simulink model "mdaqdemo_external_mode"  (R2014a)
settings: Solver=FixedStepDiscrete  SolverMode=SingleTasking  StartTime=0.0  StopTime=inf  FixedStep=0.001  RelTol=1e-3
libraries: simulink x2, microdaq_lib x2
settings Model: SimulationMode=external  CovSFcnEnable=on  ExtModeTrigDuration=10000  Creator=peselnikmg  LastModifiedBy=skibool
settings DataIOCC: SignalLoggingSaveFormat=ModelDataLogs
settings OptimizationCC: OptimizeModelRefInitCode=on  LifeSpan=1
settings DebuggingCC: UnderspecifiedInitializationDetection=Classic  MultiTaskDSMMsg=warning  MultiTaskCondExecSysMsg=none  FrameProcessingCompatibilityMsg=error  StateNameClashWarn=warning
settings HardwareCC: ProdBitPerLong=40  ProdLargestAtomicInteger=Integer  ProdIntDivRoundTo=Zero  ProdEndianess=LittleEndian  ProdHWDeviceType=Texas Instruments->C6000
settings RTWCC: SystemTargetFile=microdaq.tlc  TemplateMakefile=microdaq.tmf  PostCodeGenCommand=microdaq_postcodegen(buildInfo)  Description=MicroDAQ Real-Time Measurement System  GenerateReport=on  IncludeHyperlinkInReport=on
settings CodeAppCC: IgnoreCustomStorageClasses=off
settings STFCustomTargetCC: CodeReplacementLibrary=C89/C90 (ANSI)  ConcurrentExecutionCompliant=off  GeneratePreprocessorConditionals=Use local settings  CombineOutputUpdateFcns=on  ERTCustomFileBanners=on  SupportContinuousTime=off  SupportNonInlinedSFcns=off  MATLABClassNameForMDSCustomization=Simulink.SoftwareTarget.ERTCustomization  GRTInterface=off  SystemTargetFile=microdaq.tlc
settings ERTTargetCC: CodeReplacementLibrary=C89/C90 (ANSI)  GenerateSampleERTMain=off  ExtMode=on  ExtModeMexArgs=getpref('microdaq','TargetIP') 1 4344  InlinedParameterPlacement=Hierarchical  ERTCustomFileTemplate=microdaq_main.tlc

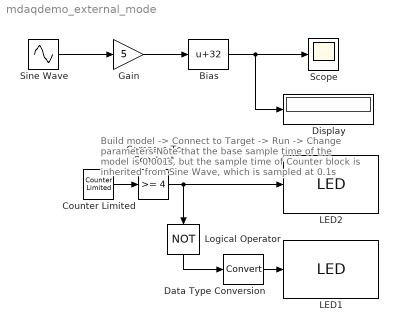
== system mdaqdemo_external_mode ==
  note: Build model -> Connect to Target -> Run -> Change parameters
      |
      | Note that the base sample time of the model is 0.001s,
      | but the sample time of Counter block is inherited from Sine Wave,
      | which is sampled at 0.1s
  Bias : Bias  Bias=32
  Compare To Constant : simulink/Logic and Bit Operations/Compare To Constant  relop=>=  const=4  OutDataTypeStr=uint8
  Counter Limited : simulink/Sources/Counter Limited  uplimit=7  tsamp=-1
      settings: AttributesFormatString=Upper limit: %<uplimit>
  Data Type Conversion : DataTypeConversion
  Display : Display
  Gain : Gain  Gain=5
  LED1 : microdaq_lib/Utilities/LED  SParameter1=D2
  LED2 : microdaq_lib/Utilities/LED  SParameter1=D1
  Logical Operator : Logic  Operator=NOT  AllPortsSameDT=off  OutDataTypeStr=boolean
  Scope : Scope
      settings: TimeRange=10  MaxDataPoints=10  SaveToWorkspace=off  SaveName=ScopeData  YMin=19.63475  YMax=44.48405  SampleTime=-1
  Sine Wave : Sin  SampleTime=0.1
      settings: AttributesFormatString=Sample Time: %<SampleTime>
  wires:
  Sine Wave/1 -> Gain/1
  Bias/1 -> Display/1, Scope/1
  Gain/1 -> Bias/1
  Compare To Constant/1 -> LED2/1, Logical Operator/1
  Logical Operator/1 -> Data Type Conversion/1
  Data Type Conversion/1 -> LED1/1
  Counter Limited/1 -> Compare To Constant/1
